simulink model "Lecture9Exercise"  (R2020b)
settings: Solver=VariableStepAuto  StartTime=0.0  StopTime=10.0  RelTol=1e-3
values from neighbouring files (symbols this model uses):
  Fs = tf(1, [f1, f0])    [Lecture9Exercise.m]
  Gp = tf(2, [1 5 -6])    [Lecture9Exercise.m]
  Hs = tf([h1, h0], 1)    [Lecture9Exercise.m]
settings Model: Creator=sebastian  LastModifiedBy=sebastian

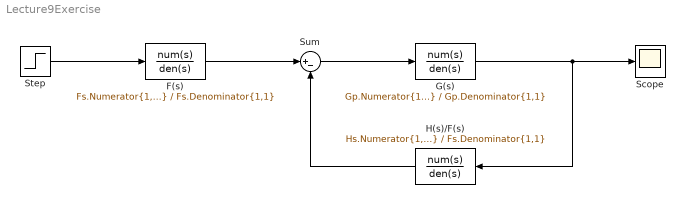
== system Lecture9Exercise ==
  F(s) : TransferFcn  Numerator=Fs.Numerator{1,1}  Denominator=Fs.Denominator{1,1}
  G(s) : TransferFcn  Numerator=Gp.Numerator{1,1}  Denominator=Gp.Denominator{1,1}
  H(s)/F(s) : TransferFcn  Numerator=Hs.Numerator{1,1}  Denominator=Fs.Denominator{1,1}
  Scope : Scope
  Step : Step  SampleTime=0
  Sum : Sum  Inputs=|+-
  wires:
  G(s)/1 -> Scope/1, H(s)/F(s)/1
  H(s)/F(s)/1 -> Sum/2
  Sum/1 -> G(s)/1
  Step/1 -> F(s)/1
  F(s)/1 -> Sum/1
